simulink model "ObserverTest"  (R2020a)
settings: Solver=FixedStepAuto  StartTime=0.0  StopTime=Sim.time  FixedStep=1e-3  MaxStep=Sim.maxStepSize  RelTol=1e-6  EnableMultiTasking=on
undefined symbols (not defined in the file or in its folder): amESO, amRESO, Controller, Plant, RefSig, Sensor
libraries: commnoisgen2 x1, simulink x1
settings Model: Creator=412  LastModifiedBy=krzychu
settings DataIOCC: ReturnWorkspaceOutputs=off  TimeSaveName=t
settings OptimizationCC: LifeSpan=inf
settings DebuggingCC: AllowSymbolicDim=off  SFUnexpectedBacktrackingDiag=warning  SFNoUnconditionalDefaultTransitionDiag=warning  SFExecutionAtInitializationDiag=none  ArithmeticOperatorsInVariantConditions=warning
settings ModelReferenceCC: PropagateSignalLabelsOutOfModel=off
settings SFSimCC: SimUseLocalCustomCode=off  CustomCodeUndefinedFunction=UseInterfaceOnly
settings RTWCC: RTWUseLocalCustomCode=off
settings CodeAppCC: StateflowObjectComments=on
settings GRTTargetCC: TargetLangStandard=C89/C90 (ANSI)
settings ConfigComp: CovMetricSettings=dw  CovHtmlReporting=on  CovSaveCumulativeToWorkspaceVar=on  CovSaveSingleToWorkspaceVar=on  CovExternalEMLEnable=off

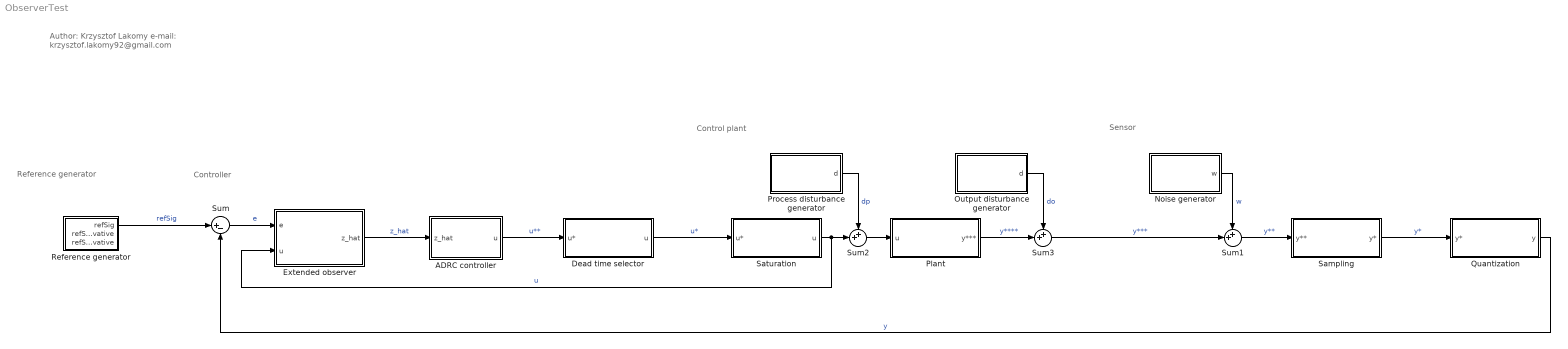
== system ObserverTest ==
  note: Author: Krzysztof Lakomy
      | e-mail: krzysztof.lakomy92@gmail.com
  note: Sensor
  note: Reference generator
  note: Controller
  note: Control plant
  ADRC controller : Subsystem
  Dead time selector : Subsystem  Variant=on
  Extended observer : Subsystem  Variant=on
  Noise generator : Subsystem  Variant=on
  Output disturbance generator : Subsystem  Variant=on
  Plant : Subsystem  Variant=on
  Process disturbance generator : Subsystem  Variant=on
  Quantization : Subsystem  Variant=on
  Reference generator : Subsystem
  Sampling : Subsystem  Variant=on
  Saturation : Subsystem  Variant=on
  Sum : Sum  Inputs=|+-
  Sum1 : Sum  Inputs=++|
  Sum2 : Sum  Inputs=++|
  Sum3 : Sum  Inputs=++|
  wires:
  Sum/1 -> Extended observer/1(e)  "e"
  Extended observer/1(z_hat) -> ADRC controller/1(z_hat)  "z_hat"
  ADRC controller/1(u) -> Dead time selector/1(u*)  "u**"
  Reference generator/1(refSig) -> Sum/1  "refSig"
  Sum1/1 -> Sampling/1(y**)  "y**"
  Noise generator/1(w) -> Sum1/1  "w"
  Sampling/1(y*) -> Quantization/1(y*)  "y*"
  Quantization/1(y) -> Sum/2  "y"
  Dead time selector/1(u) -> Saturation/1(u*)  "u*"
  Plant/1(y***) -> Sum3/2  "y****"
  Saturation/1(u) -> Extended observer/2(u), Sum2/2  "u"
  Sum2/1 -> Plant/1(u)
  Process disturbance generator/1(d) -> Sum2/1  "dp"
  Output disturbance generator/1(d) -> Sum3/1  "do"
  Sum3/1 -> Sum1/2  "y***"

== system ObserverTest/ADRC controller ==
  z_hat : Inport
  Interpreted MATLAB Function1 : MATLABFcn  MATLABFcn=adrc
  u : Outport  VectorParamsAs1DForOutWhenUnconnected=off
  wires:
  z_hat/1 -> Interpreted MATLAB Function1/1
  Interpreted MATLAB Function1/1 -> u/1  "u"

== system ObserverTest/Dead time selector ==
  u* : Inport
  Dead time off : Subsystem  VariantControl=DEADTIME_OFF
  Dead time on : Subsystem  VariantControl=DEADTIME_ON
  u : Outport  VectorParamsAs1DForOutWhenUnconnected=off

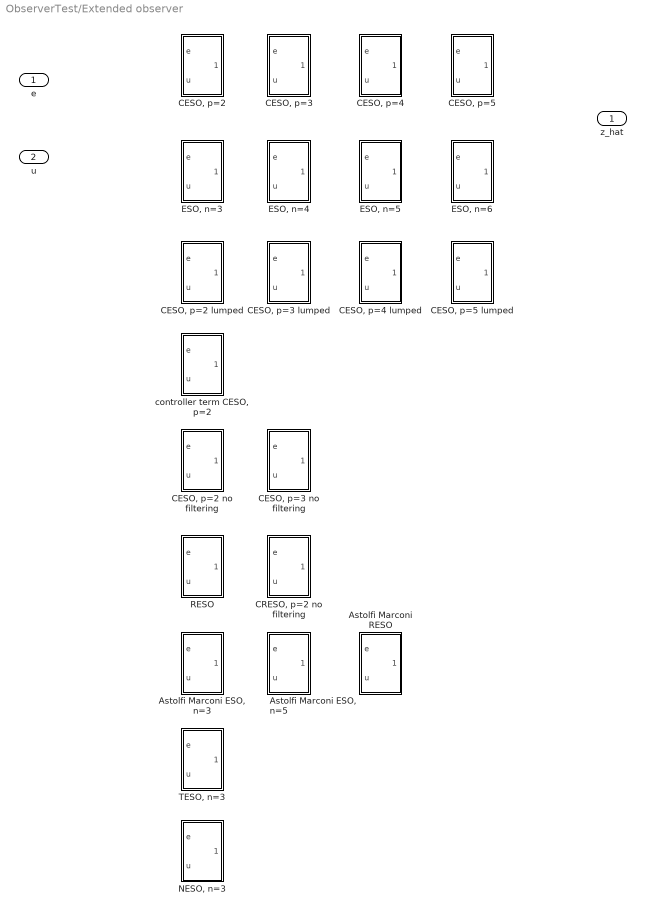
== system ObserverTest/Extended observer ==
  e : Inport
  u : Inport  Port=2
  "Astolfi Marconi ESO, n=5" : Subsystem  VariantControl=ASTOLFI_MARCONI_ESO_N5
  "Astolfi Marconi ESO, n=3" : Subsystem  VariantControl=ASTOLFI_MARCONI_ESO_N3
  Astolfi Marconi RESO : Subsystem  VariantControl=ASTOLFI_MARCONI_RESO
  "CESO, p=2" : Subsystem  VariantControl=NEW_ESO_OBSERVER_N2
  "CESO, p=2 no filtering" : Subsystem  VariantControl=CESO_NO_FILTERING_P2
  "CESO, p=2 lumped" : Subsystem  VariantControl=LUMPED_CESO_P2
  "CESO, p=3" : Subsystem  VariantControl=NEW_ESO_OBSERVER_N3
  "CESO, p=3 no filtering" : Subsystem  VariantControl=CESO_NO_FILTERING_P3
  "CESO, p=3 lumped" : Subsystem  VariantControl=LUMPED_CESO_P3
  "CESO, p=4" : Subsystem  VariantControl=NEW_ESO_OBSERVER_N4
  "CESO, p=4 lumped" : Subsystem  VariantControl=LUMPED_CESO_P4
  "CESO, p=5" : Subsystem  VariantControl=NEW_ESO_OBSERVER_N5
  "CESO, p=5 lumped" : Subsystem  VariantControl=LUMPED_CESO_P5
  "CRESO, p=2 no filtering" : Subsystem  VariantControl=CRESO_P2
  "ESO, n=3" : Subsystem  VariantControl=ESO_OBSERVER
  "ESO, n=4" : Subsystem  VariantControl=ESO_OBSERVER_N4
  "ESO, n=5" : Subsystem  VariantControl=ESO_OBSERVER_N5
  "ESO, n=6" : Subsystem  VariantControl=ESO_OBSERVER_N6
  "NESO, n=3" : Subsystem  VariantControl=NESO_N3
  RESO : Subsystem  VariantControl=RESO_N5
  "TESO, n=3" : Subsystem  VariantControl=TESO_N3
  "controller term CESO, p=2" : Subsystem  VariantControl=CONTROLLER_TERM_CESO_P2
  z_hat : Outport  VectorParamsAs1DForOutWhenUnconnected=off

== system ObserverTest/Noise generator ==
  Gaussian noise on : Subsystem  VariantControl=SENSOR_GAUSSIAN_NOISE_ON
  Noise off : Subsystem  VariantControl=SENSOR_NOISE_OFF
  White Noise on : Subsystem  VariantControl=SENSOR_WHITE_NOISE_ON
  w : Outport  VectorParamsAs1DForOutWhenUnconnected=off

== system ObserverTest/Output disturbance generator ==
  Disturbance off : Subsystem  VariantControl=OUTPUT_DISTURBANCE_OFF
  Disturbance on : Subsystem  VariantControl=OUTPUT_DISTURBANCE_ON
  d : Outport  VectorParamsAs1DForOutWhenUnconnected=off

== system ObserverTest/Plant ==
  u : Inport
  DCDC buck converter : Subsystem  VariantControl=DCDC_BUCK_CONVERTER
  Suspension ball : Subsystem  VariantControl=SUSPENSION_BALL
  transferFunction : Subsystem  VariantControl=TRANSFER_FUNCTION
  transferFunctionTimeVarying : Subsystem  VariantControl=TRANSFER_FUNCTION_TIME_VARYING
  y*** : Outport  VectorParamsAs1DForOutWhenUnconnected=off

== system ObserverTest/Process disturbance generator ==
  Disturbance off : Subsystem  VariantControl=PROCESS_DISTURBANCE_OFF
  Disturbance on : Subsystem  VariantControl=PROCESS_DISTURBANCE_ON
  d : Outport  VectorParamsAs1DForOutWhenUnconnected=off

== system ObserverTest/Quantization ==
  y* : Inport
  Quantization_off : Subsystem  VariantControl=SENSOR_QUANTIZATION_OFF
  Quantization_on : Subsystem  VariantControl=SENSOR_QUANTIZATION_ON
  y : Outport  VectorParamsAs1DForOutWhenUnconnected=off

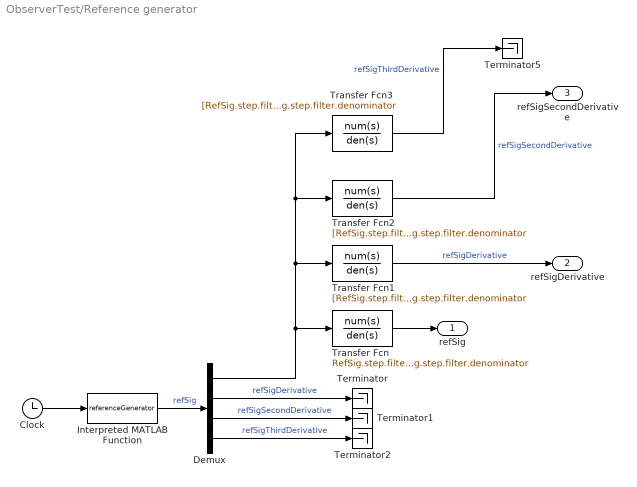
== system ObserverTest/Reference generator ==
  Clock : Clock
  Demux : Demux
  Interpreted MATLAB Function : MATLABFcn  MATLABFcn=referenceGenerator  OutputDimensions=4
  Terminator{,1..2,5} (4 alike) : Terminator
  Transfer Fcn : TransferFcn  Numerator=RefSig.step.filter.numerator  Denominator=RefSig.step.filter.denominator
  Transfer Fcn1 : TransferFcn  Numerator=[RefSig.step.filter.numerator 0]  Denominator=RefSig.step.filter.denominator
  Transfer Fcn2 : TransferFcn  Numerator=[RefSig.step.filter.numerator 0 0]  Denominator=RefSig.step.filter.denominator
  Transfer Fcn3 : TransferFcn  Numerator=[RefSig.step.filter.numerator 0 0 0]  Denominator=RefSig.step.filter.denominator
  refSig : Outport  VectorParamsAs1DForOutWhenUnconnected=off
  refSigDerivative : Outport  Port=2  VectorParamsAs1DForOutWhenUnconnected=off
  refSigSecondDerivative : Outport  Port=3  VectorParamsAs1DForOutWhenUnconnected=off
  wires:
  Clock/1 -> Interpreted MATLAB Function/1
  Interpreted MATLAB Function/1 -> Demux/1  "refSig"
  Demux/2 -> Terminator/1  "refSigDerivative"
  Demux/3 -> Terminator1/1  "refSigSecondDerivative"
  Demux/4 -> Terminator2/1  "refSigThirdDerivative"
  Demux/1 -> Transfer Fcn3/1, Transfer Fcn2/1, Transfer Fcn1/1, Transfer Fcn/1
  Transfer Fcn/1 -> refSig/1
  Transfer Fcn2/1 -> refSigSecondDerivative/1  "refSigSecondDerivative"
  Transfer Fcn1/1 -> refSigDerivative/1  "refSigDerivative"
  Transfer Fcn3/1 -> Terminator5/1  "refSigThirdDerivative"

== system ObserverTest/Sampling ==
  y** : Inport
  Sampling_off : Subsystem  VariantControl=SENSOR_SAMPLING_OFF
  Sampling_on : Subsystem  VariantControl=SENSOR_SAMPLING_ON
  y* : Outport  VectorParamsAs1DForOutWhenUnconnected=off

== system ObserverTest/Saturation ==
  u* : Inport
  Saturation off : Subsystem  VariantControl=CONTROL_SIGNAL_SATURATION_OFF
  Saturation on : Subsystem  VariantControl=CONTROL_SIGNAL_SATURATION_ON
  u : Outport  VectorParamsAs1DForOutWhenUnconnected=off

== system ObserverTest/Dead time selector/Dead time off ==
  u* : Inport
  u : Outport  VectorParamsAs1DForOutWhenUnconnected=off
  wires:
  u*/1 -> u/1

== system ObserverTest/Dead time selector/Dead time on ==
  u* : Inport
  Product : Product
  Step : Step  Time=Controller.deadTime.time  SampleTime=0
  u : Outport  VectorParamsAs1DForOutWhenUnconnected=off
  wires:
  u*/1 -> Product/1
  Step/1 -> Product/2
  Product/1 -> u/1

== system ObserverTest/Extended observer/Astolfi Marconi ESO, n=5 ==
  e : Inport
  u : Inport  Port=2
  Gain : Gain  Gain=amESO.Ln5  Multiplication=Matrix(K*u)
  Integrator1 : Integrator  InitialCondition=[0 0 0 0 0 0 0 0]'
  Interpreted MATLAB Function1 : MATLABFcn  MATLABFcn=astolfiMarconiEsoN5
  Mux1 : Mux
  z_hat : Outport  VectorParamsAs1DForOutWhenUnconnected=off
  wires:
  Integrator1/1 -> Mux1/2, Gain/1
  u/1 -> Mux1/4
  e/1 -> Mux1/3
  Mux1/1 -> Interpreted MATLAB Function1/1
  Interpreted MATLAB Function1/1 -> Integrator1/1
  Gain/1 -> Mux1/1, z_hat/1

== system ObserverTest/Extended observer/Astolfi Marconi ESO, n=3 ==
  e : Inport
  u : Inport  Port=2
  Gain : Gain  Gain=amESO.Ln3  Multiplication=Matrix(K*u)
  Integrator1 : Integrator  InitialCondition=[0 0 0 0]'
  Interpreted MATLAB Function1 : MATLABFcn  MATLABFcn=astolfiMarconiEsoN3
  Mux1 : Mux
  z_hat : Outport  VectorParamsAs1DForOutWhenUnconnected=off
  wires:
  Integrator1/1 -> Mux1/2, Gain/1
  u/1 -> Mux1/4
  e/1 -> Mux1/3
  Mux1/1 -> Interpreted MATLAB Function1/1
  Interpreted MATLAB Function1/1 -> Integrator1/1
  Gain/1 -> Mux1/1, z_hat/1

== system ObserverTest/Extended observer/Astolfi Marconi RESO ==
  e : Inport
  u : Inport  Port=2
  Gain : Gain  Gain=amRESO.L  Multiplication=Matrix(K*u)
  Integrator1 : Integrator  InitialCondition=[0 0 0 0 0 0 0 0]'
  Interpreted MATLAB Function1 : MATLABFcn  MATLABFcn=astolfiMarconiReso
  Mux1 : Mux
  z_hat : Outport  VectorParamsAs1DForOutWhenUnconnected=off
  wires:
  Integrator1/1 -> Mux1/2, Gain/1
  u/1 -> Mux1/4
  e/1 -> Mux1/3
  Mux1/1 -> Interpreted MATLAB Function1/1
  Interpreted MATLAB Function1/1 -> Integrator1/1
  Gain/1 -> Mux1/1, z_hat/1

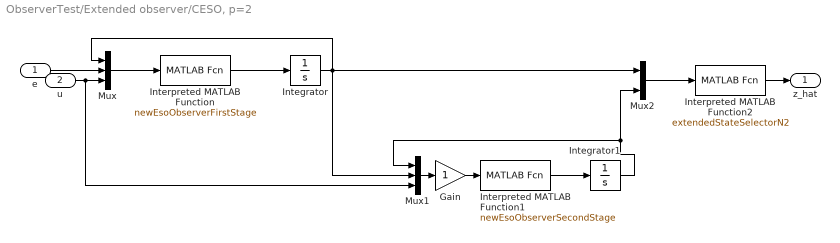
== system ObserverTest/Extended observer/CESO, p=2 ==
  e : Inport
  u : Inport  Port=2
  Gain : Gain
  Integrator : Integrator  InitialCondition=[0 0 0]'
  Integrator1 : Integrator  InitialCondition=[0 0 0]'
  Interpreted MATLAB Function : MATLABFcn  MATLABFcn=newEsoObserverFirstStage  OutputDimensions=3
  Interpreted MATLAB Function1 : MATLABFcn  MATLABFcn=newEsoObserverSecondStage  OutputDimensions=3
  Interpreted MATLAB Function2 : MATLABFcn  MATLABFcn=extendedStateSelectorN2  OutputDimensions=3
  Mux : Mux  Inputs=3
  Mux1 : Mux  Inputs=3
  Mux2 : Mux  Inputs=2
  z_hat : Outport  VectorParamsAs1DForOutWhenUnconnected=off
  wires:
  Integrator/1 -> Mux2/1, Mux/1, Mux1/2
  Mux/1 -> Interpreted MATLAB Function/1
  e/1 -> Mux/2
  u/1 -> Mux1/3, Mux/3
  Interpreted MATLAB Function/1 -> Integrator/1
  Interpreted MATLAB Function1/1 -> Integrator1/1
  Integrator1/1 -> Mux1/1, Mux2/2
  Interpreted MATLAB Function2/1 -> z_hat/1
  Mux2/1 -> Interpreted MATLAB Function2/1
  Mux1/1 -> Gain/1
  Gain/1 -> Interpreted MATLAB Function1/1

== system ObserverTest/Extended observer/CESO, p=2 no filtering ==
  e : Inport
  u : Inport  Port=2
  Integrator : Integrator  InitialCondition=zeros(6,1)
  Interpreted MATLAB Function : MATLABFcn  MATLABFcn=cesoObserverNoFilteringP2  OutputDimensions=6
  Interpreted MATLAB Function2 : MATLABFcn  MATLABFcn=extendedStateSelectorN2  OutputDimensions=3
  Mux : Mux  Inputs=3
  z_hat : Outport  VectorParamsAs1DForOutWhenUnconnected=off
  wires:
  Integrator/1 -> Interpreted MATLAB Function2/1, Mux/1
  Mux/1 -> Interpreted MATLAB Function/1
  e/1 -> Mux/2
  u/1 -> Mux/3
  Interpreted MATLAB Function/1 -> Integrator/1
  Interpreted MATLAB Function2/1 -> z_hat/1

== system ObserverTest/Extended observer/CESO, p=2 lumped ==
  e : Inport
  u : Inport  Port=2
  Integrator : Integrator  InitialCondition=zeros(6,1)
  Interpreted MATLAB Function : MATLABFcn  MATLABFcn=cesoObserverP2  OutputDimensions=6
  Interpreted MATLAB Function2 : MATLABFcn  MATLABFcn=extendedStateSelectorN2  OutputDimensions=3
  Mux : Mux  Inputs=3
  z_hat : Outport  VectorParamsAs1DForOutWhenUnconnected=off
  wires:
  Integrator/1 -> Interpreted MATLAB Function2/1, Mux/1
  Mux/1 -> Interpreted MATLAB Function/1
  e/1 -> Mux/2
  u/1 -> Mux/3
  Interpreted MATLAB Function/1 -> Integrator/1
  Interpreted MATLAB Function2/1 -> z_hat/1

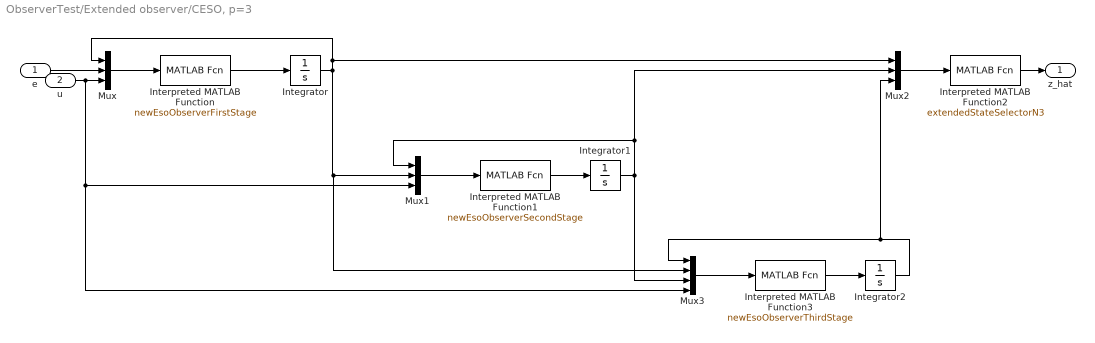
== system ObserverTest/Extended observer/CESO, p=3 ==
  e : Inport
  u : Inport  Port=2
  Integrator : Integrator  InitialCondition=[0 0 0]'
  Integrator1 : Integrator  InitialCondition=[0 0 0]'
  Integrator2 : Integrator  InitialCondition=[0 0 0]'
  Interpreted MATLAB Function : MATLABFcn  MATLABFcn=newEsoObserverFirstStage  OutputDimensions=3
  Interpreted MATLAB Function1 : MATLABFcn  MATLABFcn=newEsoObserverSecondStage  OutputDimensions=3
  Interpreted MATLAB Function2 : MATLABFcn  MATLABFcn=extendedStateSelectorN3  OutputDimensions=3
  Interpreted MATLAB Function3 : MATLABFcn  MATLABFcn=newEsoObserverThirdStage  OutputDimensions=3
  Mux : Mux  Inputs=3
  Mux1 : Mux  Inputs=3
  Mux2 : Mux  Inputs=3
  Mux3 : Mux
  z_hat : Outport  VectorParamsAs1DForOutWhenUnconnected=off
  wires:
  Integrator/1 -> Mux2/1, Mux/1, Mux3/2, Mux1/2
  Mux/1 -> Interpreted MATLAB Function/1
  e/1 -> Mux/2
  u/1 -> Mux3/4, Mux1/3, Mux/3
  Interpreted MATLAB Function/1 -> Integrator/1
  Interpreted MATLAB Function1/1 -> Integrator1/1
  Integrator1/1 -> Mux3/3, Mux1/1, Mux2/2
  Interpreted MATLAB Function2/1 -> z_hat/1
  Mux2/1 -> Interpreted MATLAB Function2/1
  Mux1/1 -> Interpreted MATLAB Function1/1
  Integrator2/1 -> Mux2/3, Mux3/1
  Mux3/1 -> Interpreted MATLAB Function3/1
  Interpreted MATLAB Function3/1 -> Integrator2/1

== system ObserverTest/Extended observer/CESO, p=3 no filtering ==
  e : Inport
  u : Inport  Port=2
  Integrator : Integrator  InitialCondition=zeros(9,1)
  Interpreted MATLAB Function : MATLABFcn  MATLABFcn=cesoObserverNoFilteringP3  OutputDimensions=9
  Interpreted MATLAB Function2 : MATLABFcn  MATLABFcn=extendedStateSelectorN3  OutputDimensions=3
  Mux : Mux  Inputs=3
  z_hat : Outport  VectorParamsAs1DForOutWhenUnconnected=off
  wires:
  Integrator/1 -> Interpreted MATLAB Function2/1, Mux/1
  Mux/1 -> Interpreted MATLAB Function/1
  e/1 -> Mux/2
  u/1 -> Mux/3
  Interpreted MATLAB Function/1 -> Integrator/1
  Interpreted MATLAB Function2/1 -> z_hat/1

== system ObserverTest/Extended observer/CESO, p=3 lumped ==
  e : Inport
  u : Inport  Port=2
  Integrator : Integrator  InitialCondition=zeros(9,1)
  Interpreted MATLAB Function : MATLABFcn  MATLABFcn=cesoObserverP3  OutputDimensions=9
  Interpreted MATLAB Function2 : MATLABFcn  MATLABFcn=extendedStateSelectorN3  OutputDimensions=3
  Mux : Mux  Inputs=3
  z_hat : Outport  VectorParamsAs1DForOutWhenUnconnected=off
  wires:
  Integrator/1 -> Interpreted MATLAB Function2/1, Mux/1
  Mux/1 -> Interpreted MATLAB Function/1
  e/1 -> Mux/2
  u/1 -> Mux/3
  Interpreted MATLAB Function/1 -> Integrator/1
  Interpreted MATLAB Function2/1 -> z_hat/1

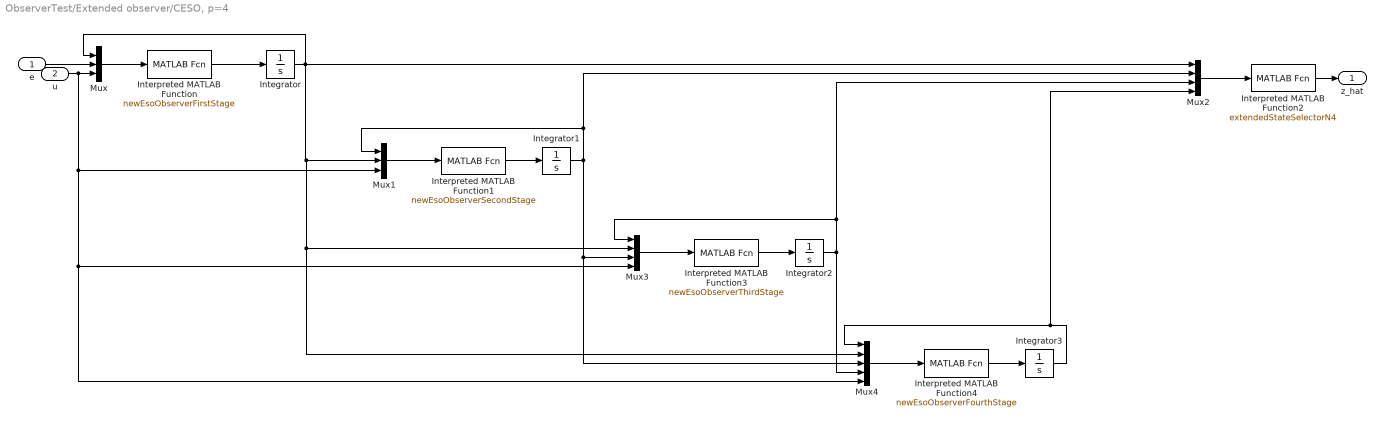
== system ObserverTest/Extended observer/CESO, p=4 ==
  e : Inport
  u : Inport  Port=2
  Integrator{,1..3} (4 alike) : Integrator  InitialCondition=[0 0 0]'
  Interpreted MATLAB Function : MATLABFcn  MATLABFcn=newEsoObserverFirstStage  OutputDimensions=3
  Interpreted MATLAB Function1 : MATLABFcn  MATLABFcn=newEsoObserverSecondStage  OutputDimensions=3
  Interpreted MATLAB Function2 : MATLABFcn  MATLABFcn=extendedStateSelectorN4  OutputDimensions=3
  Interpreted MATLAB Function3 : MATLABFcn  MATLABFcn=newEsoObserverThirdStage  OutputDimensions=3
  Interpreted MATLAB Function4 : MATLABFcn  MATLABFcn=newEsoObserverFourthStage  OutputDimensions=3
  Mux : Mux  Inputs=3
  Mux1 : Mux  Inputs=3
  Mux2 : Mux
  Mux3 : Mux
  Mux4 : Mux  Inputs=5
  z_hat : Outport  VectorParamsAs1DForOutWhenUnconnected=off
  wires:
  Integrator/1 -> Mux/1, Mux2/1, Mux4/2, Mux3/2, Mux1/2
  Mux/1 -> Interpreted MATLAB Function/1
  e/1 -> Mux/2
  u/1 -> Mux4/5, Mux3/4, Mux1/3, Mux/3
  Interpreted MATLAB Function/1 -> Integrator/1
  Interpreted MATLAB Function1/1 -> Integrator1/1
  Integrator1/1 -> Mux3/3, Mux4/3, Mux1/1, Mux2/2
  Interpreted MATLAB Function2/1 -> z_hat/1
  Mux2/1 -> Interpreted MATLAB Function2/1
  Mux1/1 -> Interpreted MATLAB Function1/1
  Integrator2/1 -> Mux4/4, Mux3/1, Mux2/3
  Mux3/1 -> Interpreted MATLAB Function3/1
  Interpreted MATLAB Function3/1 -> Integrator2/1
  Mux4/1 -> Interpreted MATLAB Function4/1
  Integrator3/1 -> Mux2/4, Mux4/1
  Interpreted MATLAB Function4/1 -> Integrator3/1

== system ObserverTest/Extended observer/CESO, p=4 lumped ==
  e : Inport
  u : Inport  Port=2
  Integrator : Integrator  InitialCondition=zeros(12,1)
  Interpreted MATLAB Function : MATLABFcn  MATLABFcn=cesoObserverP4  OutputDimensions=12
  Interpreted MATLAB Function2 : MATLABFcn  MATLABFcn=extendedStateSelectorN4  OutputDimensions=3
  Mux : Mux  Inputs=3
  z_hat : Outport  VectorParamsAs1DForOutWhenUnconnected=off
  wires:
  Integrator/1 -> Interpreted MATLAB Function2/1, Mux/1
  Mux/1 -> Interpreted MATLAB Function/1
  e/1 -> Mux/2
  u/1 -> Mux/3
  Interpreted MATLAB Function/1 -> Integrator/1
  Interpreted MATLAB Function2/1 -> z_hat/1

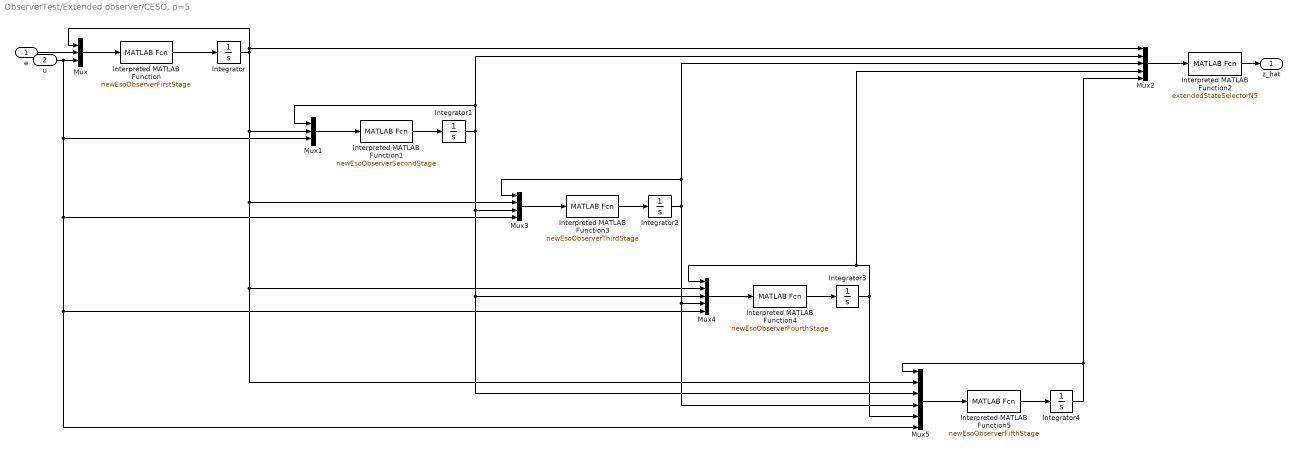
== system ObserverTest/Extended observer/CESO, p=5 ==
  e : Inport
  u : Inport  Port=2
  Integrator{,1..4} (5 alike) : Integrator  InitialCondition=[0 0 0]'
  Interpreted MATLAB Function : MATLABFcn  MATLABFcn=newEsoObserverFirstStage  OutputDimensions=3
  Interpreted MATLAB Function1 : MATLABFcn  MATLABFcn=newEsoObserverSecondStage  OutputDimensions=3
  Interpreted MATLAB Function2 : MATLABFcn  MATLABFcn=extendedStateSelectorN5  OutputDimensions=3
  Interpreted MATLAB Function3 : MATLABFcn  MATLABFcn=newEsoObserverThirdStage  OutputDimensions=3
  Interpreted MATLAB Function4 : MATLABFcn  MATLABFcn=newEsoObserverFourthStage  OutputDimensions=3
  Interpreted MATLAB Function5 : MATLABFcn  MATLABFcn=newEsoObserverFifthStage  OutputDimensions=3
  Mux : Mux  Inputs=3
  Mux1 : Mux  Inputs=3
  Mux2 : Mux  Inputs=5
  Mux3 : Mux
  Mux4 : Mux  Inputs=5
  Mux5 : Mux  Inputs=6
  z_hat : Outport  VectorParamsAs1DForOutWhenUnconnected=off
  wires:
  Integrator/1 -> Mux/1, Mux2/1, Mux4/2, Mux5/2, Mux3/2, Mux1/2
  Mux/1 -> Interpreted MATLAB Function/1
  e/1 -> Mux/2
  u/1 -> Mux5/6, Mux4/5, Mux3/4, Mux1/3, Mux/3
  Interpreted MATLAB Function/1 -> Integrator/1
  Interpreted MATLAB Function1/1 -> Integrator1/1
  Integrator1/1 -> Mux3/3, Mux5/3, Mux4/3, Mux1/1, Mux2/2
  Interpreted MATLAB Function2/1 -> z_hat/1
  Mux2/1 -> Interpreted MATLAB Function2/1
  Mux1/1 -> Interpreted MATLAB Function1/1
  Integrator2/1 -> Mux5/4, Mux4/4, Mux3/1, Mux2/3
  Mux3/1 -> Interpreted MATLAB Function3/1
  Interpreted MATLAB Function3/1 -> Integrator2/1
  Mux4/1 -> Interpreted MATLAB Function4/1
  Integrator3/1 -> Mux2/4, Mux4/1, Mux5/5
  Interpreted MATLAB Function4/1 -> Integrator3/1
  Integrator4/1 -> Mux5/1, Mux2/5
  Mux5/1 -> Interpreted MATLAB Function5/1
  Interpreted MATLAB Function5/1 -> Integrator4/1

== system ObserverTest/Extended observer/CESO, p=5 lumped ==
  e : Inport
  u : Inport  Port=2
  Integrator : Integrator  InitialCondition=zeros(15,1)
  Interpreted MATLAB Function : MATLABFcn  MATLABFcn=cesoObserverP5  OutputDimensions=15
  Interpreted MATLAB Function2 : MATLABFcn  MATLABFcn=extendedStateSelectorN5  OutputDimensions=3
  Mux : Mux  Inputs=3
  z_hat : Outport  VectorParamsAs1DForOutWhenUnconnected=off
  wires:
  Integrator/1 -> Interpreted MATLAB Function2/1, Mux/1
  Mux/1 -> Interpreted MATLAB Function/1
  e/1 -> Mux/2
  u/1 -> Mux/3
  Interpreted MATLAB Function/1 -> Integrator/1
  Interpreted MATLAB Function2/1 -> z_hat/1

== system ObserverTest/Extended observer/CRESO, p=2 no filtering ==
  e : Inport
  u : Inport  Port=2
  Integrator : Integrator  InitialCondition=zeros(10,1)
  Interpreted MATLAB Function : MATLABFcn  MATLABFcn=cresoObserverP2  OutputDimensions=10
  Interpreted MATLAB Function2 : MATLABFcn  MATLABFcn=cresoExtendedStateSelectorN2  OutputDimensions=3
  Mux : Mux  Inputs=3
  z_hat : Outport  VectorParamsAs1DForOutWhenUnconnected=off
  wires:
  Integrator/1 -> Interpreted MATLAB Function2/1, Mux/1
  Mux/1 -> Interpreted MATLAB Function/1
  e/1 -> Mux/2
  u/1 -> Mux/3
  Interpreted MATLAB Function/1 -> Integrator/1
  Interpreted MATLAB Function2/1 -> z_hat/1

== system ObserverTest/Extended observer/ESO, n=3 ==
  e : Inport
  u : Inport  Port=2
  Integrator : Integrator  InitialCondition=[0 0 0]'
  Interpreted MATLAB Function : MATLABFcn  MATLABFcn=esoObserver  OutputDimensions=3
  Mux : Mux  Inputs=3
  z_hat : Outport  VectorParamsAs1DForOutWhenUnconnected=off
  wires:
  Integrator/1 -> z_hat/1, Mux/1
  Mux/1 -> Interpreted MATLAB Function/1
  e/1 -> Mux/2
  u/1 -> Mux/3
  Interpreted MATLAB Function/1 -> Integrator/1

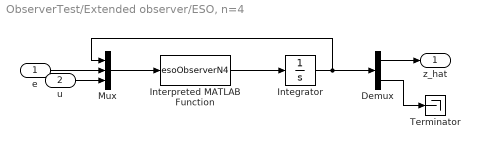
== system ObserverTest/Extended observer/ESO, n=4 ==
  e : Inport
  u : Inport  Port=2
  Demux : Demux  Outputs=[3 1]
  Integrator : Integrator  InitialCondition=[0 0 0 0]'
  Interpreted MATLAB Function : MATLABFcn  MATLABFcn=esoObserverN4  OutputDimensions=4
  Mux : Mux  Inputs=3
  Terminator : Terminator
  z_hat : Outport  VectorParamsAs1DForOutWhenUnconnected=off
  wires:
  Integrator/1 -> Demux/1, Mux/1
  Mux/1 -> Interpreted MATLAB Function/1
  e/1 -> Mux/2
  u/1 -> Mux/3
  Interpreted MATLAB Function/1 -> Integrator/1
  Demux/1 -> z_hat/1
  Demux/2 -> Terminator/1

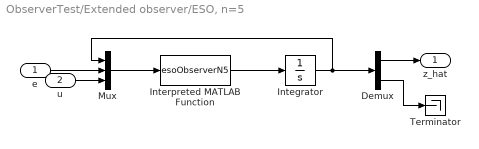
== system ObserverTest/Extended observer/ESO, n=5 ==
  e : Inport
  u : Inport  Port=2
  Demux : Demux  Outputs=[3 2]
  Integrator : Integrator  InitialCondition=[0 0 0 0 0]'
  Interpreted MATLAB Function : MATLABFcn  MATLABFcn=esoObserverN5  OutputDimensions=5
  Mux : Mux  Inputs=3
  Terminator : Terminator
  z_hat : Outport  VectorParamsAs1DForOutWhenUnconnected=off
  wires:
  Integrator/1 -> Demux/1, Mux/1
  Mux/1 -> Interpreted MATLAB Function/1
  e/1 -> Mux/2
  u/1 -> Mux/3
  Interpreted MATLAB Function/1 -> Integrator/1
  Demux/1 -> z_hat/1
  Demux/2 -> Terminator/1

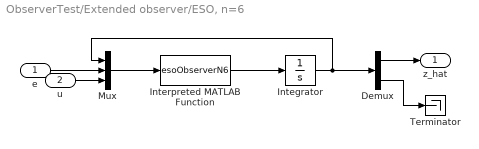
== system ObserverTest/Extended observer/ESO, n=6 ==
  e : Inport
  u : Inport  Port=2
  Demux : Demux  Outputs=[3 3]
  Integrator : Integrator  InitialCondition=[0 0 0 0 0 0]'
  Interpreted MATLAB Function : MATLABFcn  MATLABFcn=esoObserverN6  OutputDimensions=6
  Mux : Mux  Inputs=3
  Terminator : Terminator
  z_hat : Outport  VectorParamsAs1DForOutWhenUnconnected=off
  wires:
  Integrator/1 -> Demux/1, Mux/1
  Mux/1 -> Interpreted MATLAB Function/1
  e/1 -> Mux/2
  u/1 -> Mux/3
  Interpreted MATLAB Function/1 -> Integrator/1
  Demux/1 -> z_hat/1
  Demux/2 -> Terminator/1

== system ObserverTest/Extended observer/NESO, n=3 ==
  e : Inport
  u : Inport  Port=2
  Integrator : Integrator  InitialCondition=[0 0 0]'
  Interpreted MATLAB Function : MATLABFcn  MATLABFcn=nesoObserver  OutputDimensions=3
  Mux : Mux  Inputs=3
  z_hat : Outport  VectorParamsAs1DForOutWhenUnconnected=off
  wires:
  Integrator/1 -> z_hat/1, Mux/1
  Mux/1 -> Interpreted MATLAB Function/1
  e/1 -> Mux/2
  u/1 -> Mux/3
  Interpreted MATLAB Function/1 -> Integrator/1

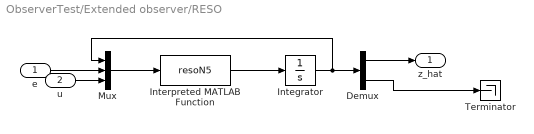
== system ObserverTest/Extended observer/RESO ==
  e : Inport
  u : Inport  Port=2
  Demux : Demux  Outputs=[3 2]
  Integrator : Integrator  InitialCondition=[0 0 0 0 0]'
  Interpreted MATLAB Function : MATLABFcn  MATLABFcn=resoN5  OutputDimensions=5
  Mux : Mux  Inputs=3
  Terminator : Terminator
  z_hat : Outport  VectorParamsAs1DForOutWhenUnconnected=off
  wires:
  Integrator/1 -> Demux/1, Mux/1
  Mux/1 -> Interpreted MATLAB Function/1
  e/1 -> Mux/2
  u/1 -> Mux/3
  Interpreted MATLAB Function/1 -> Integrator/1
  Demux/1 -> z_hat/1
  Demux/2 -> Terminator/1

== system ObserverTest/Extended observer/TESO, n=3 ==
  e : Inport
  u : Inport  Port=2
  Clock : Clock
  Integrator : Integrator  InitialCondition=[0 0 0]'
  Interpreted MATLAB Function : MATLABFcn  MATLABFcn=esoObserver  OutputDimensions=3
  Mux : Mux
  z_hat : Outport  VectorParamsAs1DForOutWhenUnconnected=off
  wires:
  Integrator/1 -> z_hat/1, Mux/1
  Mux/1 -> Interpreted MATLAB Function/1
  e/1 -> Mux/2
  u/1 -> Mux/3
  Interpreted MATLAB Function/1 -> Integrator/1
  Clock/1 -> Mux/4

== system ObserverTest/Extended observer/controller term CESO, p=2 ==
  e : Inport
  u : Inport  Port=2
  Integrator : Integrator  InitialCondition=zeros(6,1)
  Interpreted MATLAB Function : MATLABFcn  MATLABFcn=controllerTermCesoObserverP2  OutputDimensions=6
  Interpreted MATLAB Function2 : MATLABFcn  MATLABFcn=extendedStateSelectorN2  OutputDimensions=3
  Mux : Mux  Inputs=3
  z_hat : Outport  VectorParamsAs1DForOutWhenUnconnected=off
  wires:
  Integrator/1 -> Interpreted MATLAB Function2/1, Mux/1
  Mux/1 -> Interpreted MATLAB Function/1
  e/1 -> Mux/2
  u/1 -> Mux/3
  Interpreted MATLAB Function/1 -> Integrator/1
  Interpreted MATLAB Function2/1 -> z_hat/1

== system ObserverTest/Noise generator/Gaussian noise on ==
  Gain2 : Gain  Gain=Sensor.gaussianNoise.gain
  Gaussian Noise Generator : commnoisgen2/Gaussian Noise Generator  m=Sensor.gaussianNoise.meanValue  d=Sensor.gaussianNoise.variance  s=Sensor.gaussianNoise.initialSeed  Ts=Sensor.gaussianNoise.sampleTime  frameBased=off  sampPerFrame=1  orient=off  outDataType=double
      settings: SourceProductBaseCode=CM
  w : Outport  VectorParamsAs1DForOutWhenUnconnected=off
  wires:
  Gain2/1 -> w/1  "w"
  Gaussian Noise Generator/1 -> Gain2/1

== system ObserverTest/Noise generator/Noise off ==
  Constant : Constant  Value=0
  w : Outport  VectorParamsAs1DForOutWhenUnconnected=off
  wires:
  Constant/1 -> w/1

== system ObserverTest/Noise generator/White Noise on ==
  Band-Limited White Noise : simulink/Sources/Band-Limited White Noise  Cov=Sensor.whiteNoise.power  Ts=Sensor.whiteNoise.Ts  seed=Sensor.whiteNoise.seed
  w : Outport  VectorParamsAs1DForOutWhenUnconnected=off
  wires:
  Band-Limited White Noise/1 -> w/1  "w"

== system ObserverTest/Output disturbance generator/Disturbance off ==
  Constant : Constant  Value=0
  d : Outport  VectorParamsAs1DForOutWhenUnconnected=off
  wires:
  Constant/1 -> d/1

== system ObserverTest/Output disturbance generator/Disturbance on ==
  Clock : Clock
  Interpreted MATLAB Function : MATLABFcn  MATLABFcn=outputDisturbanceGenerator
  d : Outport  VectorParamsAs1DForOutWhenUnconnected=off
  wires:
  Clock/1 -> Interpreted MATLAB Function/1
  Interpreted MATLAB Function/1 -> d/1  "d"

== system ObserverTest/Plant/DCDC buck converter ==
  u : Inport
  Gain : Gain  Gain=Plant.dcdcBuckConverter.C  Multiplication=Matrix(K*u)
  Integrator : Integrator  InitialCondition=Plant.dcdcBuckConverter.x0
  Interpreted MATLAB Function : MATLABFcn  MATLABFcn=dcdcBuckConverter
  Mux : Mux  Inputs=2
  y*** : Outport  VectorParamsAs1DForOutWhenUnconnected=off
  wires:
  u/1 -> Mux/2
  Gain/1 -> y***/1  "y**"
  Mux/1 -> Interpreted MATLAB Function/1
  Interpreted MATLAB Function/1 -> Integrator/1  "xp"
  Integrator/1 -> Mux/1, Gain/1  "x"

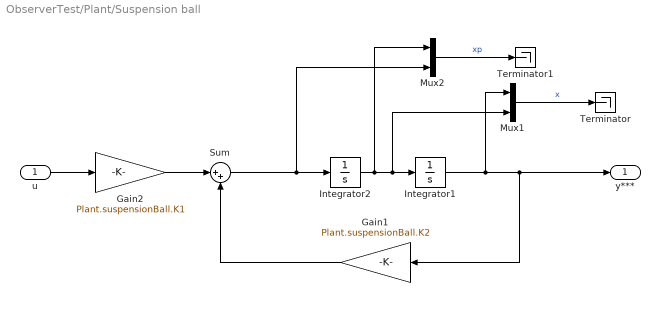
== system ObserverTest/Plant/Suspension ball ==
  u : Inport
  Gain1 : Gain  Gain=Plant.suspensionBall.K2
  Gain2 : Gain  Gain=Plant.suspensionBall.K1
  Integrator1 : Integrator  InitialCondition=Plant.suspensionBall.x0(1)
  Integrator2 : Integrator  InitialCondition=Plant.suspensionBall.x0(2)
  Mux1 : Mux  Inputs=2
  Mux2 : Mux  Inputs=2
  Sum : Sum  Inputs=|++
  Terminator : Terminator
  Terminator1 : Terminator
  y*** : Outport  VectorParamsAs1DForOutWhenUnconnected=off
  wires:
  u/1 -> Gain2/1
  Gain1/1 -> Sum/2
  Gain2/1 -> Sum/1
  Integrator1/1 -> Mux1/1, y***/1, Gain1/1
  Mux1/1 -> Terminator/1  "x"
  Mux2/1 -> Terminator1/1  "xp"
  Sum/1 -> Mux2/2, Integrator2/1
  Integrator2/1 -> Mux2/1, Mux1/2, Integrator1/1

== system ObserverTest/Plant/transferFunction ==
  u : Inport
  Gain : Gain  Gain=Plant.transferFunction.C  Multiplication=Matrix(K*u)
  Integrator : Integrator  InitialCondition=Plant.transferFunction.x0
  Interpreted MATLAB Function : MATLABFcn  MATLABFcn=transferFunction
  Mux : Mux  Inputs=2
  y*** : Outport  VectorParamsAs1DForOutWhenUnconnected=off
  wires:
  u/1 -> Mux/2
  Gain/1 -> y***/1  "y**"
  Mux/1 -> Interpreted MATLAB Function/1
  Interpreted MATLAB Function/1 -> Integrator/1  "xp"
  Integrator/1 -> Mux/1, Gain/1  "x"

== system ObserverTest/Plant/transferFunctionTimeVarying ==
  u : Inport
  Clock : Clock
  Gain : Gain  Gain=Plant.transferFunction.C  Multiplication=Matrix(K*u)
  Integrator : Integrator  InitialCondition=Plant.transferFunction.x0
  Interpreted MATLAB Function : MATLABFcn  MATLABFcn=transferFunctionTimeVarying
  Mux : Mux  Inputs=3
  y*** : Outport  VectorParamsAs1DForOutWhenUnconnected=off
  wires:
  u/1 -> Mux/2
  Gain/1 -> y***/1  "y**"
  Mux/1 -> Interpreted MATLAB Function/1
  Interpreted MATLAB Function/1 -> Integrator/1  "xp"
  Integrator/1 -> Mux/1, Gain/1  "x"
  Clock/1 -> Mux/3

== system ObserverTest/Process disturbance generator/Disturbance off ==
  Constant : Constant  Value=0
  d : Outport  VectorParamsAs1DForOutWhenUnconnected=off
  wires:
  Constant/1 -> d/1

== system ObserverTest/Process disturbance generator/Disturbance on ==
  Clock : Clock
  Interpreted MATLAB Function : MATLABFcn  MATLABFcn=processDisturbanceGenerator
  d : Outport  VectorParamsAs1DForOutWhenUnconnected=off
  wires:
  Clock/1 -> Interpreted MATLAB Function/1
  Interpreted MATLAB Function/1 -> d/1  "d"

== system ObserverTest/Quantization/Quantization_off ==
  y* : Inport
  y : Outport  VectorParamsAs1DForOutWhenUnconnected=off
  wires:
  y*/1 -> y/1

== system ObserverTest/Quantization/Quantization_on ==
  y* : Inport
  Quantizer : Quantizer  QuantizationInterval=Sensor.quantization.interval
  y : Outport  VectorParamsAs1DForOutWhenUnconnected=off
  wires:
  y*/1 -> Quantizer/1
  Quantizer/1 -> y/1

== system ObserverTest/Sampling/Sampling_off ==
  y** : Inport
  y* : Outport  VectorParamsAs1DForOutWhenUnconnected=off
  wires:
  y**/1 -> y*/1

== system ObserverTest/Sampling/Sampling_on ==
  y** : Inport
  Rate Transition1 : RateTransition  OutPortSampleTime=Sensor.sampling.rate
  y* : Outport  VectorParamsAs1DForOutWhenUnconnected=off
  wires:
  y**/1 -> Rate Transition1/1
  Rate Transition1/1 -> y*/1

== system ObserverTest/Saturation/Saturation off ==
  u* : Inport
  u : Outport  VectorParamsAs1DForOutWhenUnconnected=off
  wires:
  u*/1 -> u/1

== system ObserverTest/Saturation/Saturation on ==
  u* : Inport
  Saturation : Saturate  UpperLimit=Plant.controlSignalSaturation.upperLimit  LowerLimit=Plant.controlSignalSaturation.lowerLimit
  u : Outport  VectorParamsAs1DForOutWhenUnconnected=off
  wires:
  u*/1 -> Saturation/1
  Saturation/1 -> u/1
